simulink subsystem "AtmosphericDrag_SS"  (R2023a)
settings: Solver=VariableStepAuto  StartTime=0.0  StopTime=10.0  RelTol=1e-3
settings Model: Creator=jself  LastModifiedBy=willb

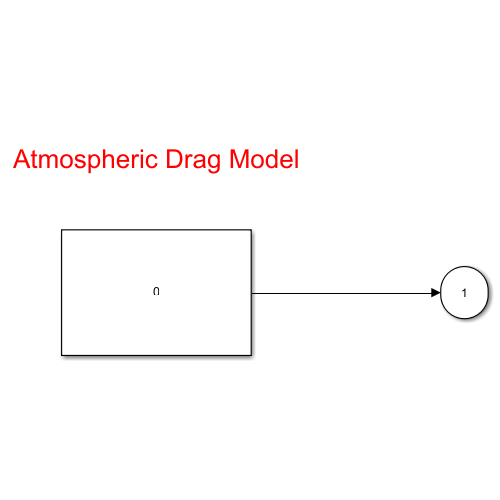
[thumbnail: Simulink's stored preview of the top-level diagram]
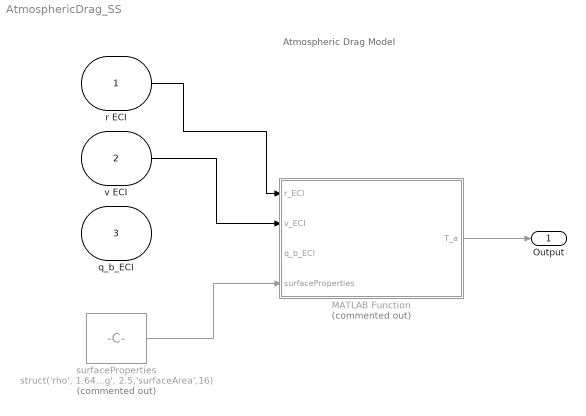
== system AtmosphericDrag_SS ==
  note: Atmospheric Drag Model
  r ECI : Inport
  v ECI : Inport  Port=2
  q_b_ECI : Inport  Port=3
  MATLAB Function : MATLAB Function  Commented=on  TreatAsAtomicUnit=on
  surfaceProperties : Constant  Commented=on  Value=struct('rho', 1.647454703531699e-14, 'drag', 2.5,'surfaceArea',16)  LockScale=on
  Output : Outport
  wires:
  MATLAB Function/1(T_a) -> Output/1
  surfaceProperties/1 -> MATLAB Function/4(surfaceProperties)
  v ECI/1 -> MATLAB Function/2(v_ECI)
  r ECI/1 -> MATLAB Function/1(r_ECI)

== matlab function AtmosphericDrag_SS/MATLAB Function ==
  data: T_a output; r_ECI input; v_ECI input; q_b_ECI input; surfaceProperties input
function T_a = aero_drag_torque(r_ECI, v_ECI, q_b_ECI, surfaceProperties)

% Calculate aerodynamic torque 
% bringing in drag coe and rho 
% a_wet in ram direction -- body x added 
% center of pressure 


Cd = surfaceProperties.drag;
A = surfaceProperties.surfaceArea; %taking body x direction measurements ! 
rho = surfaceProperties.rho;

v_rel_ECI = v_ECI - cross(r_ECI, q_b_ECI);
v_rel_mag = norm(v_rel_ECI);

% Use rho? 
T_a = -0.5 * Cd * A * v_rel_mag^2 * cross(v_rel_ECI, q_b_ECI);

end
